simulink model "PVAndBatteryIntegratedPlantForBlackStart"  (R2025b)
settings: Solver=FixedStepAuto  StartTime=0.0  StopTime=tsim  FixedStep=1e-6  RelTol=1e-9  AbsTol=1e-7
InitFcn:
  | %% Black Start Sequence
  | t0 = 0; % Battery IBR initial time
  | t1 = 0.15; % PV IBR initial time
  | t2 = 0.5; % Two IBR sync time
  | t3 = 0.8; % Additional motor load connect
  | t4 = 1.1; % Grid reconnection
  | tsim = 1.5; % Total simulation time
  | 
  | %% initialize
  | Vdc = 400;
  | Vnom = 100;
  | Prated = 10000;
  | Qrated = 0;
  | Srated = sqrt(Prated^2+Qrated^2);
  | wnom = 2*pi*60;
  | fnom = 60;
  | Vminpu = 0.95;
  | 
  | kv = Vnom;
  | ki = 3*Vnom/Srated;
  | 
  | dwmax = 0.5*2*pi;
  | trisemax = 0.1;
  | 
  | C = 1/sqrt(2)/Vminpu^2/dwmax;
  | L = 1/C/wnom^2;
  | tau = C/kv/ki;
  | epsilon = sqrt(L/C);
  | ksy = 3/2/trisemax;
  | 
  | V_voc_1 = 0;
  | V_voc_2 = 0;
  | 
  | % filter
  | Rf = 0.05;
  | Lf = 500e-6;
  | % pwm
  | fsw = 10e3;
  | % simulation
  | Ts = 1e-6;
  | 
  | % load
  | Rl = 3*Vnom^2/Prated;
  | Rl1 = Rl;
  | Rl2 = 2*Rl;
  | Rl3 = 20*Rl;
  | % grid
  | Rg = 0.05;
  | Lg = 50e-6;
  | 
  | % DCDC converter
  | Kp_V = 1;
  | Ki_V = 0.02;
  | Imax = 110;
  | Kp_I = 0.0001;
  | Ki_I = 1;
  | Vcmax = 1;
undefined symbols (not defined in the file): alpha, C_voc, Diode_class, Half_BridgeConverter_class, L_voc, Ll, Mosfet_class, PWMGenerator_DC_DC__class, R_voc, Three_PhaseBreaker_class, Three_PhaseSource_class, Three_PhaseTransformer_2_class, Three_PhaseV_IMeasuremen_class
libraries: nesl_utility x69, ee_lib x49, fl_lib x36, mcbeeMathTransformLib x9, simulink x6, spsParallelRLCBranchLib x3, eePwmGeneratorTwoLevel x2, spsControlledCurrentSourceLib x2, elec_conv_HighZElecRef x2, slpidlib x2, spsSecondOrderFilterLib x1, spsCurrentMeasurementLib x1
(part 3 of 4)

== system PVAndBatteryIntegratedPlantForBlackStart/PV Inverter /PV Array ==
  S : Inport
  TempC : Inport  Port=2
  CSns : fl_lib/Electrical/Electrical Sensors/Current Sensor
  SC : ee_lib/Sources/Solar Cell  prm=ee.enum.sources.solar_cell_prm.datasheet  Isc=11.31 A  Voc=0.66071 V  Is=1e-6 A  Is2=0 A  Iph=11.31 A  Ir0=1000 W/m^2  ec=1.5  N2=2  Rs=0.0033987 Ohm  Rp=2.559 Ohm  N_series=280  N_parallel=10  TIPH1=0 1/K  EG=1.11 eV  TXIS1=3  TXIS2=3  TRS1=0  TRP1=0  Tmeas=25 degC  TFIXED=25 degC  thermal_mass=100 J/K  initial_temperature=25 degC
  VSns : fl_lib/Electrical/Electrical Sensors/Voltage Sensor
  busM : BusCreator  Inputs=2
  i2s : nesl_utility/PS-Simulink Converter  PhysicalDomain=network_engine_domain  SubClassName=ps_output  LeftPortType=input  RightPortType=output  PseudoPeriodic=off  Frequencies=[]  VectorFormat=inherit  Unit=inherit  AffineConversion=off
  s2ps : nesl_utility/Simulink-PS Converter  PhysicalDomain=network_engine_domain  SubClassName=ps_input  LeftPortType=input  RightPortType=output  PseudoPeriodic=off  Frequencies=[]  NoiseDistribution=none  NoiseParameters=[]  Unit=W/m^2  AffineConversion=off  FilteringAndDerivatives=provide  SimscapeFilterOrder=1  InputFilterTimeConstant=0.001  UdotUserProvided=0
  termT : Terminator
  v2s : nesl_utility/PS-Simulink Converter  PhysicalDomain=network_engine_domain  SubClassName=ps_output  LeftPortType=input  RightPortType=output  PseudoPeriodic=off  Frequencies=[]  VectorFormat=inherit  Unit=inherit  AffineConversion=off
  + : PMIOPort  Side=Right
  - : PMIOPort  Port=2  Side=Right
  m : Outport  VectorParamsAs1DForOutWhenUnconnected=off
  wires:
  S/1 -> s2ps/1
  TempC/1 -> termT/1
  v2s/1 -> busM/1  "V_PV"
  busM/1 -> m/1
  i2s/1 -> busM/2  "I_PV"
  connections:
  CSns/RConn1 -- i2s/LConn1
  VSns/RConn1 -- v2s/LConn1
  CSns/RConn2 -- +/RConn1
  VSns/RConn2 -- SC/RConn1 -- -/RConn1
  s2ps/RConn1 -- SC/LConn1
  VSns/LConn1 -- SC/LConn2 -- CSns/LConn1

== system PVAndBatteryIntegratedPlantForBlackStart/PV Inverter /PWM Generator (DC-DC) ==
  D : Inport
  PWM Generator : eePwmGenerator/PWM Generator  CarrCount=Up  Tper=PWMGenerator_DC_DC__class(fsw).objParamMappingDerived.NewDerivedParam.Tper  Tdelay=0  Ts=Ts
  P : Outport  VectorParamsAs1DForOutWhenUnconnected=off
  wires:
  D/1 -> PWM Generator/1
  PWM Generator/1 -> P/1

== system PVAndBatteryIntegratedPlantForBlackStart/PV Inverter /Series RLC Branch ==
  Inductor : fl_lib/Electrical/Electrical Elements/Inductor  l=0.0006 H  r=0 Ohm  g=1e-9 1/Ohm  i_specify=off  i_priority=None  i=0 A  i_nominal_specify=off  i_nominal_value=1  i_nominal_unit=A  v_specify=off  v_priority=None  v=0 V  v_nominal_specify=off  v_nominal_value=1  v_nominal_unit=V  i_L_specify=on  i_L_priority=None  i_L=0 A  i_L_nominal_specify=off  i_L_nominal_value=1  i_L_nominal_unit=A
  Resistor : fl_lib/Electrical/Electrical Elements/Resistor  R=0.001 Ohm  i_specify=off  i_priority=None  i=0 A  i_nominal_specify=off  i_nominal_value=1  i_nominal_unit=A  v_specify=off  v_priority=None  v=0 V  v_nominal_specify=off  v_nominal_value=1  v_nominal_unit=V
  + : PMIOPort  Side=Left
  - : PMIOPort  Port=2  Side=Right
  connections:
  Inductor/LConn1 -- Resistor/RConn1
  +/RConn1 -- Resistor/LConn1
  Inductor/RConn1 -- -/RConn1

== system PVAndBatteryIntegratedPlantForBlackStart/PV Inverter /Series RLC Branch1 ==
  Capacitor : fl_lib/Electrical/Electrical Elements/Capacitor  c=0.01 F  r=1e-6 Ohm  g=0 1/Ohm  i_specify=off  i_priority=None  i=0 A  i_nominal_specify=off  i_nominal_value=1  i_nominal_unit=A  v_specify=off  v_priority=None  v=0 V  v_nominal_specify=off  v_nominal_value=1  v_nominal_unit=V  vc_specify=on  vc_priority=High  vc=Vdc V  vc_nominal_specify=off  vc_nominal_value=1  vc_nominal_unit=V
  Resistor : fl_lib/Electrical/Electrical Elements/Resistor  R=0.001 Ohm  i_specify=off  i_priority=None  i=0 A  i_nominal_specify=off  i_nominal_value=1  i_nominal_unit=A  v_specify=off  v_priority=None  v=0 V  v_nominal_specify=off  v_nominal_value=1  v_nominal_unit=V
  + : PMIOPort  Side=Left
  - : PMIOPort  Port=2  Side=Right
  connections:
  Capacitor/RConn1 -- -/RConn1
  +/RConn1 -- Resistor/LConn1
  Resistor/RConn1 -- Capacitor/LConn1

== system PVAndBatteryIntegratedPlantForBlackStart/PV Inverter /Series RLC Branch2 ==
  Capacitor : fl_lib/Electrical/Electrical Elements/Capacitor  c=0.001 F  r=1e-6 Ohm  g=0 1/Ohm  i_specify=off  i_priority=None  i=0 A  i_nominal_specify=off  i_nominal_value=1  i_nominal_unit=A  v_specify=off  v_priority=None  v=0 V  v_nominal_specify=off  v_nominal_value=1  v_nominal_unit=V  vc_specify=on  vc_priority=None  vc=0 V  vc_nominal_specify=off  vc_nominal_value=1  vc_nominal_unit=V
  Resistor : fl_lib/Electrical/Electrical Elements/Resistor  R=0.001 Ohm  i_specify=off  i_priority=None  i=0 A  i_nominal_specify=off  i_nominal_value=1  i_nominal_unit=A  v_specify=off  v_priority=None  v=0 V  v_nominal_specify=off  v_nominal_value=1  v_nominal_unit=V
  + : PMIOPort  Side=Left
  - : PMIOPort  Port=2  Side=Right
  connections:
  Capacitor/RConn1 -- -/RConn1
  +/RConn1 -- Resistor/LConn1
  Resistor/RConn1 -- Capacitor/LConn1

== system PVAndBatteryIntegratedPlantForBlackStart/PV Inverter /Three-Phase Breaker ==
  Circuit Breaker : ee_lib/Switches & Breakers/Circuit Breaker (Three-Phase)  R_closed=0.001 Ohm  G_open=Three_PhaseBreaker_class('open',1000000,Inf,t1,'off').objParamMappingDerived.NewDerivedParam.G_open 1/Ohm  threshold=0.5 V  breaker_behavior=ee.enum.switches.breakerBehavior.zeroCrossingEnable
      settings: InternalSimscapePortConfiguration="{\"Bottom\":[],\"Left\":[{\"id\":\"vT\",\"label\":\"vT\",\"type\":\"input\"},{\"id\":\"a1\",\"label\":\"a1\",\"type\":\"foundation.electrical.electrical\"},{\"id\":\"b1\",\"label\":\"b1\",\"type\":\"foundation.electrical.electrical\"},{\"id\":\"c1\",\"label\":\"c1\",\"type\":\"foundation.electrical.electrical\"}],\"Right\":[{\"id\":\"a2\",\"label\":\"a2\",\"type\":\"foundation.electrical.electrical\"},{\"id\":\"b2\",\"label\":\"b2\",\"type\":\"foundation.electrical.electrical\"},{\"id\":\"c2\",\"label\":\"c2\",\"type\":\"foundation.electrical.electrical\"}],\"Top\":[]}"
  com : Subsystem
  A : PMIOPort  Side=Left
  B : PMIOPort  Port=2  Side=Left
  C : PMIOPort  Port=3  Side=Left
  a : PMIOPort  Port=4  Side=Right
  b : PMIOPort  Port=5  Side=Right
  c : PMIOPort  Port=6  Side=Right
  connections:
  Circuit Breaker/LConn1 -- com/RConn1
  Circuit Breaker/LConn2 -- A/RConn1
  Circuit Breaker/LConn3 -- B/RConn1
  Circuit Breaker/LConn4 -- C/RConn1
  Circuit Breaker/RConn1 -- a/RConn1
  Circuit Breaker/RConn2 -- b/RConn1
  Circuit Breaker/RConn3 -- c/RConn1

== system PVAndBatteryIntegratedPlantForBlackStart/PV Inverter /VOC Control ==
  Ifb : Inport
  P : Inport  Port=2
  Q : Inport  Port=3
  Constant : Constant  Value=0
  Inverse Clarke Transform : mcbeeMathTransformLib/Inverse Clarke Transform  PowerInvariant=off  UseWithEmbedded=off  PhaseInput=Two inputs
      settings: LibrarySourceBlock=|
      | ee_sl_lib/Mathematical
      | Transforms/Inverse
      | Clarke Transform
  Memory : Memory
  Memory1 : Memory
  Mux1 : Mux  Inputs=3
  Mux2 : Mux  Inputs=2
  Scope2 : Scope  NumInputPorts=6
      settings: ActiveDisplayYMinimum=-1297.23542  ActiveDisplayYMaximum=1334.98027
  Subsystem : Subsystem
  VOC_DE : Subsystem
  Vref : Outport
  tag scope: V_albe_inv_2=global
  wires:
  Mux2/1 -> [V_albe_inv_2]
  Q/1 -> Subsystem/3(Q)
  P/1 -> Subsystem/2(P)
  Subsystem/1(u) -> VOC_DE/1(u), Scope2/2
  Constant/1 -> Mux1/3
  VOC_DE/2(vbe) -> Memory1/1, Mux2/2, Mux1/2, Scope2/4
  VOC_DE/1(val) -> Mux1/1, Scope2/3, Memory/1, Mux2/1
  Inverse Clarke Transform/1 -> Scope2/6, Vref/1
  Ifb/1 -> Scope2/1, Subsystem/1(If)
  Mux1/1 -> Inverse Clarke Transform/1, Scope2/5
  Memory/1 -> Subsystem/4(val)
  Memory1/1 -> Subsystem/5(vbe)

== system PVAndBatteryIntegratedPlantForBlackStart/PV Inverter /Voltage Measurement ==
  PS-Simulink Converter : nesl_utility/PS-Simulink Converter  PhysicalDomain=network_engine_domain  SubClassName=ps_output  LeftPortType=input  RightPortType=output  PseudoPeriodic=off  Frequencies=[]  VectorFormat=1-D array  Unit=V  AffineConversion=off
  Voltage Sensor : fl_lib/Electrical/Electrical Sensors/Voltage Sensor
  + : PMIOPort  Side=Left
  - : PMIOPort  Port=2  Side=Left
  v : Outport  VectorParamsAs1DForOutWhenUnconnected=off
  wires:
  PS-Simulink Converter/1 -> v/1
  connections:
  PS-Simulink Converter/LConn1 -- Voltage Sensor/RConn1
  -/RConn1 -- Voltage Sensor/RConn2
  +/RConn1 -- Voltage Sensor/LConn1

== system PVAndBatteryIntegratedPlantForBlackStart/PV Inverter /inv ==
  Current and Voltage Sensor (Three-Phase) : ee_lib/Sensors & Transducers/Current and Voltage Sensor (Three-Phase)  vMeasurementType=2  outputUnit=2  SRated=100000000 V*A  VRated=500000 V  I_specify=off  I_priority=None  I=[ 0 0 0 ] A  I_nominal_specify=off  I_nominal_value=1  I_nominal_unit=A  V_specify=off  V_priority=None  V=[ 0 0 0 ] V  V_nominal_specify=off  V_nominal_value=1  V_nominal_unit=V
      settings: InternalSimscapePortConfiguration="{\"Bottom\":[],\"Left\":[{\"id\":\"a1\",\"label\":\"a1\",\"type\":\"foundation.electrical.electrical\"},{\"id\":\"b1\",\"label\":\"b1\",\"type\":\"foundation.electrical.electrical\"},{\"id\":\"c1\",\"label\":\"c1\",\"type\":\"foundation.electrical.electrical\"}],\"Right\":[{\"id\":\"V_output\",\"label\":\"V\",\"type\":\"output\"},{\"id\":\"I_output\",\"label\":\"I\",\"type\":\"output\"},{\"id\":\"a2\",\"label\":\"a2\",\"type\":\"foundation.electrical.electrical\"},{\"id\":\"b2\",\"label\":\"b2\",\"type\":\"foundation.electrical.electrical\"},{\"id\":\"c2\",\"label\":\"c2\",\"type\":\"foundation.electrical.electrical\"}],\"Top\":[]}"
  Igain : Gain  Gain=Three_PhaseV_IMeasuremen_class('phase-to-ground','yes','off','off','off',100000000,500000).objParamMappingDerived.NewDerivedParam.IG
  PS-Simulink Converter : nesl_utility/PS-Simulink Converter  PhysicalDomain=network_engine_domain  SubClassName=ps_output  LeftPortType=input  RightPortType=output  PseudoPeriodic=off  Frequencies=[]  VectorFormat=1-D array  Unit=1  AffineConversion=off
  PS-Simulink Converter1 : nesl_utility/PS-Simulink Converter  PhysicalDomain=network_engine_domain  SubClassName=ps_output  LeftPortType=input  RightPortType=output  PseudoPeriodic=off  Frequencies=[]  VectorFormat=1-D array  Unit=1  AffineConversion=off
  Vgain : Gain  Gain=Three_PhaseV_IMeasuremen_class('phase-to-ground','yes','off','off','off',100000000,500000).objParamMappingDerived.NewDerivedParam.VG
  A : PMIOPort  Side=Left
  B : PMIOPort  Port=2  Side=Left
  C : PMIOPort  Port=3  Side=Left
  a : PMIOPort  Port=4  Side=Right
  b : PMIOPort  Port=5  Side=Right
  c : PMIOPort  Port=6  Side=Right
  Vabc : Outport  VectorParamsAs1DForOutWhenUnconnected=off
  Iabc : Outport  Port=2  VectorParamsAs1DForOutWhenUnconnected=off
  wires:
  Igain/1 -> Iabc/1
  Vgain/1 -> Vabc/1
  PS-Simulink Converter1/1 -> Igain/1
  PS-Simulink Converter/1 -> Vgain/1
  connections:
  Current and Voltage Sensor (Three-Phase)/RConn1 -- PS-Simulink Converter/LConn1
  Current and Voltage Sensor (Three-Phase)/RConn2 -- PS-Simulink Converter1/LConn1
  Current and Voltage Sensor (Three-Phase)/RConn5 -- c/RConn1
  Current and Voltage Sensor (Three-Phase)/RConn4 -- b/RConn1
  Current and Voltage Sensor (Three-Phase)/RConn3 -- a/RConn1
  Current and Voltage Sensor (Three-Phase)/LConn3 -- C/RConn1
  Current and Voltage Sensor (Three-Phase)/LConn1 -- A/RConn1
  Current and Voltage Sensor (Three-Phase)/LConn2 -- B/RConn1

== system PVAndBatteryIntegratedPlantForBlackStart/PV Inverter /inv1 ==
  Current and Voltage Sensor (Three-Phase) : ee_lib/Sensors & Transducers/Current and Voltage Sensor (Three-Phase)  vMeasurementType=2  outputUnit=2  SRated=100000000 V*A  VRated=500000 V  I_specify=off  I_priority=None  I=[ 0 0 0 ] A  I_nominal_specify=off  I_nominal_value=1  I_nominal_unit=A  V_specify=off  V_priority=None  V=[ 0 0 0 ] V  V_nominal_specify=off  V_nominal_value=1  V_nominal_unit=V
      settings: InternalSimscapePortConfiguration="{\"Bottom\":[],\"Left\":[{\"id\":\"a1\",\"label\":\"a1\",\"type\":\"foundation.electrical.electrical\"},{\"id\":\"b1\",\"label\":\"b1\",\"type\":\"foundation.electrical.electrical\"},{\"id\":\"c1\",\"label\":\"c1\",\"type\":\"foundation.electrical.electrical\"}],\"Right\":[{\"id\":\"V_output\",\"label\":\"V\",\"type\":\"output\"},{\"id\":\"I_output\",\"label\":\"I\",\"type\":\"output\"},{\"id\":\"a2\",\"label\":\"a2\",\"type\":\"foundation.electrical.electrical\"},{\"id\":\"b2\",\"label\":\"b2\",\"type\":\"foundation.electrical.electrical\"},{\"id\":\"c2\",\"label\":\"c2\",\"type\":\"foundation.electrical.electrical\"}],\"Top\":[]}"
  Igain : Gain  Gain=Three_PhaseV_IMeasuremen_class('phase-to-ground','yes','off','off','off',100000000,500000).objParamMappingDerived.NewDerivedParam.IG
  PS-Simulink Converter : nesl_utility/PS-Simulink Converter  PhysicalDomain=network_engine_domain  SubClassName=ps_output  LeftPortType=input  RightPortType=output  PseudoPeriodic=off  Frequencies=[]  VectorFormat=1-D array  Unit=1  AffineConversion=off
  PS-Simulink Converter1 : nesl_utility/PS-Simulink Converter  PhysicalDomain=network_engine_domain  SubClassName=ps_output  LeftPortType=input  RightPortType=output  PseudoPeriodic=off  Frequencies=[]  VectorFormat=1-D array  Unit=1  AffineConversion=off
  Vgain : Gain  Gain=Three_PhaseV_IMeasuremen_class('phase-to-ground','yes','off','off','off',100000000,500000).objParamMappingDerived.NewDerivedParam.VG
  A : PMIOPort  Side=Left
  B : PMIOPort  Port=2  Side=Left
  C : PMIOPort  Port=3  Side=Left
  a : PMIOPort  Port=4  Side=Right
  b : PMIOPort  Port=5  Side=Right
  c : PMIOPort  Port=6  Side=Right
  Vabc : Outport  VectorParamsAs1DForOutWhenUnconnected=off
  Iabc : Outport  Port=2  VectorParamsAs1DForOutWhenUnconnected=off
  wires:
  Igain/1 -> Iabc/1
  Vgain/1 -> Vabc/1
  PS-Simulink Converter1/1 -> Igain/1
  PS-Simulink Converter/1 -> Vgain/1
  connections:
  Current and Voltage Sensor (Three-Phase)/RConn1 -- PS-Simulink Converter/LConn1
  Current and Voltage Sensor (Three-Phase)/RConn2 -- PS-Simulink Converter1/LConn1
  Current and Voltage Sensor (Three-Phase)/RConn5 -- c/RConn1
  Current and Voltage Sensor (Three-Phase)/RConn4 -- b/RConn1
  Current and Voltage Sensor (Three-Phase)/RConn3 -- a/RConn1
  Current and Voltage Sensor (Three-Phase)/LConn3 -- C/RConn1
  Current and Voltage Sensor (Three-Phase)/LConn1 -- A/RConn1
  Current and Voltage Sensor (Three-Phase)/LConn2 -- B/RConn1

== system PVAndBatteryIntegratedPlantForBlackStart/Three-Phase Breaker/com ==
  AND : Logic  Operator=NXOR  Inputs=5  IconShape=distinctive  AllPortsSameDT=off  OutDataTypeStr=boolean
  Data Type Conversion : DataTypeConversion  SaturateOnIntegerOverflow=off  RndMeth=Floor
  Simulink-PS Converter : nesl_utility/Simulink-PS Converter  PhysicalDomain=network_engine_domain  SubClassName=ps_input  LeftPortType=input  RightPortType=output  PseudoPeriodic=off  Frequencies=[]  NoiseDistribution=none  NoiseParameters=[]  Unit=1  AffineConversion=off  FilteringAndDerivatives=provide  SimscapeFilterOrder=1  InputFilterTimeConstant=0.001  UdotUserProvided=0
  Step : Step  Time=Three_PhaseBreaker_class('open',1000000,Inf,t4,'off').objParamMappingDerived.NewDerivedParam.switchTime1  SampleTime=0
  Step1 : Step  Time=Three_PhaseBreaker_class('open',1000000,Inf,t4,'off').objParamMappingDerived.NewDerivedParam.switchTime2  SampleTime=0
  Step2 : Step  Time=Three_PhaseBreaker_class('open',1000000,Inf,t4,'off').objParamMappingDerived.NewDerivedParam.switchTime3  SampleTime=0
  Step3 : Step  Time=Three_PhaseBreaker_class('open',1000000,Inf,t4,'off').objParamMappingDerived.NewDerivedParam.switchTime4  SampleTime=0
  Step4 : Step  Time=Three_PhaseBreaker_class('open',1000000,Inf,t4,'off').objParamMappingDerived.NewDerivedParam.switchTime5  SampleTime=0
  CB : PMIOPort  Side=Right
  wires:
  Data Type Conversion/1 -> Simulink-PS Converter/1
  Step4/1 -> AND/5
  AND/1 -> Data Type Conversion/1
  Step3/1 -> AND/4
  Step1/1 -> AND/2
  Step/1 -> AND/1
  Step2/1 -> AND/3
  connections:
  Simulink-PS Converter/RConn1 -- CB/RConn1

== system PVAndBatteryIntegratedPlantForBlackStart/Three-Phase Breaker1/com ==
  AND : Logic  Operator=NXOR  Inputs=5  IconShape=distinctive  AllPortsSameDT=off  OutDataTypeStr=boolean
  Data Type Conversion : DataTypeConversion  SaturateOnIntegerOverflow=off  RndMeth=Floor
  Simulink-PS Converter : nesl_utility/Simulink-PS Converter  PhysicalDomain=network_engine_domain  SubClassName=ps_input  LeftPortType=input  RightPortType=output  PseudoPeriodic=off  Frequencies=[]  NoiseDistribution=none  NoiseParameters=[]  Unit=1  AffineConversion=off  FilteringAndDerivatives=provide  SimscapeFilterOrder=1  InputFilterTimeConstant=0.001  UdotUserProvided=0
  Step : Step  Time=Three_PhaseBreaker_class('open',1000000,Inf,t2,'off').objParamMappingDerived.NewDerivedParam.switchTime1  SampleTime=0
  Step1 : Step  Time=Three_PhaseBreaker_class('open',1000000,Inf,t2,'off').objParamMappingDerived.NewDerivedParam.switchTime2  SampleTime=0
  Step2 : Step  Time=Three_PhaseBreaker_class('open',1000000,Inf,t2,'off').objParamMappingDerived.NewDerivedParam.switchTime3  SampleTime=0
  Step3 : Step  Time=Three_PhaseBreaker_class('open',1000000,Inf,t2,'off').objParamMappingDerived.NewDerivedParam.switchTime4  SampleTime=0
  Step4 : Step  Time=Three_PhaseBreaker_class('open',1000000,Inf,t2,'off').objParamMappingDerived.NewDerivedParam.switchTime5  SampleTime=0
  CB : PMIOPort  Side=Right
  wires:
  Data Type Conversion/1 -> Simulink-PS Converter/1
  Step4/1 -> AND/5
  AND/1 -> Data Type Conversion/1
  Step3/1 -> AND/4
  Step1/1 -> AND/2
  Step/1 -> AND/1
  Step2/1 -> AND/3
  connections:
  Simulink-PS Converter/RConn1 -- CB/RConn1

== system PVAndBatteryIntegratedPlantForBlackStart/Three-Phase Breaker2/com ==
  AND : Logic  Operator=NXOR  Inputs=5  IconShape=distinctive  AllPortsSameDT=off  OutDataTypeStr=boolean
  Data Type Conversion : DataTypeConversion  SaturateOnIntegerOverflow=off  RndMeth=Floor
  Simulink-PS Converter : nesl_utility/Simulink-PS Converter  PhysicalDomain=network_engine_domain  SubClassName=ps_input  LeftPortType=input  RightPortType=output  PseudoPeriodic=off  Frequencies=[]  NoiseDistribution=none  NoiseParameters=[]  Unit=1  AffineConversion=off  FilteringAndDerivatives=provide  SimscapeFilterOrder=1  InputFilterTimeConstant=0.001  UdotUserProvided=0
  Step : Step  Time=Three_PhaseBreaker_class('open',1000000000,Inf,t3,'off').objParamMappingDerived.NewDerivedParam.switchTime1  SampleTime=0
  Step1 : Step  Time=Three_PhaseBreaker_class('open',1000000000,Inf,t3,'off').objParamMappingDerived.NewDerivedParam.switchTime2  SampleTime=0
  Step2 : Step  Time=Three_PhaseBreaker_class('open',1000000000,Inf,t3,'off').objParamMappingDerived.NewDerivedParam.switchTime3  SampleTime=0
  Step3 : Step  Time=Three_PhaseBreaker_class('open',1000000000,Inf,t3,'off').objParamMappingDerived.NewDerivedParam.switchTime4  SampleTime=0
  Step4 : Step  Time=Three_PhaseBreaker_class('open',1000000000,Inf,t3,'off').objParamMappingDerived.NewDerivedParam.switchTime5  SampleTime=0
  CB : PMIOPort  Side=Right
  wires:
  Data Type Conversion/1 -> Simulink-PS Converter/1
  Step4/1 -> AND/5
  AND/1 -> Data Type Conversion/1
  Step3/1 -> AND/4
  Step1/1 -> AND/2
  Step/1 -> AND/1
  Step2/1 -> AND/3
  connections:
  Simulink-PS Converter/RConn1 -- CB/RConn1

== system PVAndBatteryIntegratedPlantForBlackStart/Three-Phase Breaker3/com ==
  AND : Logic  Operator=NXOR  Inputs=5  IconShape=distinctive  AllPortsSameDT=off  OutDataTypeStr=boolean
  Data Type Conversion : DataTypeConversion  SaturateOnIntegerOverflow=off  RndMeth=Floor
  Simulink-PS Converter : nesl_utility/Simulink-PS Converter  PhysicalDomain=network_engine_domain  SubClassName=ps_input  LeftPortType=input  RightPortType=output  PseudoPeriodic=off  Frequencies=[]  NoiseDistribution=none  NoiseParameters=[]  Unit=1  AffineConversion=off  FilteringAndDerivatives=provide  SimscapeFilterOrder=1  InputFilterTimeConstant=0.001  UdotUserProvided=0
  Step : Step  Time=Three_PhaseBreaker_class('open',1000000,Inf,t4,'off').objParamMappingDerived.NewDerivedParam.switchTime1  SampleTime=0
  Step1 : Step  Time=Three_PhaseBreaker_class('open',1000000,Inf,t4,'off').objParamMappingDerived.NewDerivedParam.switchTime2  SampleTime=0
  Step2 : Step  Time=Three_PhaseBreaker_class('open',1000000,Inf,t4,'off').objParamMappingDerived.NewDerivedParam.switchTime3  SampleTime=0
  Step3 : Step  Time=Three_PhaseBreaker_class('open',1000000,Inf,t4,'off').objParamMappingDerived.NewDerivedParam.switchTime4  SampleTime=0
  Step4 : Step  Time=Three_PhaseBreaker_class('open',1000000,Inf,t4,'off').objParamMappingDerived.NewDerivedParam.switchTime5  SampleTime=0
  CB : PMIOPort  Side=Right
  wires:
  Data Type Conversion/1 -> Simulink-PS Converter/1
  Step4/1 -> AND/5
  AND/1 -> Data Type Conversion/1
  Step3/1 -> AND/4
  Step1/1 -> AND/2
  Step/1 -> AND/1
  Step2/1 -> AND/3
  connections:
  Simulink-PS Converter/RConn1 -- CB/RConn1

== system PVAndBatteryIntegratedPlantForBlackStart/Battery Inverter/Inverter/Half-Bridge Converter ==
  " g " : Inport
  BL : Inport  Port=2
  Compare To Constant : simulink/Logic and Bit Operations/Compare To Constant  relop=<=  const=0.5  OutDataTypeStr=boolean
  Data Type Conversion : DataTypeConversion  OutDataTypeStr=double  SaturateOnIntegerOverflow=off  RndMeth=Floor
  Demux : Demux  Outputs=2
  Multiply : Product
  Simulink-PS Converter : nesl_utility/Simulink-PS Converter  PhysicalDomain=network_engine_domain  SubClassName=ps_input  LeftPortType=input  RightPortType=output  PseudoPeriodic=off  Frequencies=[]  NoiseDistribution=none  NoiseParameters=[]  Unit=1  AffineConversion=off  FilteringAndDerivatives=provide  SimscapeFilterOrder=1  InputFilterTimeConstant=0.001  UdotUserProvided=0
  Simulink-PS Converter1 : nesl_utility/Simulink-PS Converter  PhysicalDomain=network_engine_domain  SubClassName=ps_input  LeftPortType=input  RightPortType=output  PseudoPeriodic=off  Frequencies=[]  NoiseDistribution=none  NoiseParameters=[]  Unit=1  AffineConversion=off  FilteringAndDerivatives=provide  SimscapeFilterOrder=1  InputFilterTimeConstant=0.001  UdotUserProvided=0
  Two-Pulse Gate Multiplexer : ee_lib/Semiconductors & Converters/Converters/Two-Pulse Gate Multiplexer  port_option=ee.enum.controlport.ps
      settings: InternalSimscapePortConfiguration="{\"Bottom\":[],\"Left\":[{\"id\":\"G1_ps\",\"label\":\"G1\",\"type\":\"input\"},{\"id\":\"G2_ps\",\"label\":\"G2\",\"type\":\"input\"}],\"Right\":[{\"id\":\"p\",\"label\":\"G\",\"type\":\"foundation.electrical.four_phase\"}],\"Top\":[]}"
  Two-Quadrant Chopper : ee_lib/Semiconductors & Converters/Converters/Two-Quadrant Chopper  device_type=3  Vf=Half_BridgeConverter_class('Switching devices',0.001,1000000,Inf,0.001,1000000,Inf,0.001).objParamMappingDerived.NewDerivedParam.Vf V  Ron=Half_BridgeConverter_class('Switching devices',0.001,1000000,Inf,0.001,1000000,Inf,0.001).objParamMappingDerived.NewDerivedParam.Ron Ohm  Rds=0.001 Ohm  Goff=Half_BridgeConverter_class('Switching devices',0.001,1000000,Inf,0.001,1000000,Inf,0.001).objParamMappingDerived.NewDerivedParam.Goff 1/Ohm  Vgt=1 V  Vgt_off=-1 V  Ih=1 A  Vth=0.5 V  K=0  diode_param=2  diode_Vf=Half_BridgeConverter_class('Switching devices',0.001,1000000,Inf,0.001,1000000,Inf,0.001).objParamMappingDerived.NewDerivedParam.diode_Vf V  diode_Ron=Half_BridgeConverter_class('Switching devices',0.001,1000000,Inf,0.001,1000000,Inf,0.001).objParamMappingDerived.NewDerivedParam.diode_Ron Ohm  diode_Goff=Half_BridgeConverter_class('Switching devices',0.001,1000000,Inf,0.001,1000000,Inf,0.001).objParamMappingDerived.NewDerivedParam.diode_Goff 1/Ohm  diode_C=50 nF  diode_iRM=-235 A  diode_iF=300 A  diode_idot=-50 A/us  diode_trr_param=1  diode_trr_factor=3  diode_trr=15 us  diode_Qrr=1500 s*uA  snubber_type=0  Cs=Half_BridgeConverter_class('Switching devices',0.001,1000000,Inf,0.001,1000000,Inf,0.001).objParamMappingDerived.NewDerivedParam.Cs F  Rs=Half_BridgeConverter_class('Switching devices',0.001,1000000,Inf,0.001,1000000,Inf,0.001).objParamMappingDerived.NewDerivedParam.Rs Ohm
      settings: InternalSimscapePortConfiguration="{\"Bottom\":[],\"Left\":[{\"id\":\"G\",\"label\":\"G\",\"type\":\"foundation.electrical.four_phase\"},{\"id\":\"p1\",\"label\":\"1+\",\"type\":\"foundation.electrical.electrical\"},{\"id\":\"n1\",\"label\":\"1-\",\"type\":\"foundation.electrical.electrical\"}],\"Right\":[{\"id\":\"p2\",\"label\":\"2+\",\"type\":\"foundation.electrical.electrical\"},{\"id\":\"n2\",\"label\":\"2-\",\"type\":\"foundation.electrical.electrical\"}],\"Top\":[]}"
  + : PMIOPort  Side=Right
  - : PMIOPort  Port=2  Side=Right
  1 : PMIOPort  Port=3  Side=Left
  wires:
  Demux/2 -> Simulink-PS Converter1/1
  Demux/1 -> Simulink-PS Converter/1
  Multiply/1 -> Demux/1
  Data Type Conversion/1 -> Multiply/2
  Compare To Constant/1 -> Data Type Conversion/1
  BL/1 -> Compare To Constant/1
  " g "/1 -> Multiply/1
  connections:
  Simulink-PS Converter1/RConn1 -- Two-Pulse Gate Multiplexer/LConn2
  Two-Pulse Gate Multiplexer/RConn1 -- Two-Quadrant Chopper/LConn1
  Simulink-PS Converter/RConn1 -- Two-Pulse Gate Multiplexer/LConn1
  +/RConn1 -- Two-Quadrant Chopper/LConn2
  1/RConn1 -- Two-Quadrant Chopper/RConn1
  Two-Quadrant Chopper/LConn3 -- Two-Quadrant Chopper/RConn2 -- -/RConn1

== system PVAndBatteryIntegratedPlantForBlackStart/Battery Inverter/Inverter/Half-Bridge Converter1 ==
  " g " : Inport
  BL : Inport  Port=2
  Compare To Constant : simulink/Logic and Bit Operations/Compare To Constant  relop=<=  const=0.5  OutDataTypeStr=boolean
  Data Type Conversion : DataTypeConversion  OutDataTypeStr=double  SaturateOnIntegerOverflow=off  RndMeth=Floor
  Demux : Demux  Outputs=2
  Multiply : Product
  Simulink-PS Converter : nesl_utility/Simulink-PS Converter  PhysicalDomain=network_engine_domain  SubClassName=ps_input  LeftPortType=input  RightPortType=output  PseudoPeriodic=off  Frequencies=[]  NoiseDistribution=none  NoiseParameters=[]  Unit=1  AffineConversion=off  FilteringAndDerivatives=provide  SimscapeFilterOrder=1  InputFilterTimeConstant=0.001  UdotUserProvided=0
  Simulink-PS Converter1 : nesl_utility/Simulink-PS Converter  PhysicalDomain=network_engine_domain  SubClassName=ps_input  LeftPortType=input  RightPortType=output  PseudoPeriodic=off  Frequencies=[]  NoiseDistribution=none  NoiseParameters=[]  Unit=1  AffineConversion=off  FilteringAndDerivatives=provide  SimscapeFilterOrder=1  InputFilterTimeConstant=0.001  UdotUserProvided=0
  Two-Pulse Gate Multiplexer : ee_lib/Semiconductors & Converters/Converters/Two-Pulse Gate Multiplexer  port_option=ee.enum.controlport.ps
      settings: InternalSimscapePortConfiguration="{\"Bottom\":[],\"Left\":[{\"id\":\"G1_ps\",\"label\":\"G1\",\"type\":\"input\"},{\"id\":\"G2_ps\",\"label\":\"G2\",\"type\":\"input\"}],\"Right\":[{\"id\":\"p\",\"label\":\"G\",\"type\":\"foundation.electrical.four_phase\"}],\"Top\":[]}"
  Two-Quadrant Chopper : ee_lib/Semiconductors & Converters/Converters/Two-Quadrant Chopper  device_type=3  Vf=Half_BridgeConverter_class('Switching devices',0.001,1000000,Inf,0.001,1000000,Inf,0.001).objParamMappingDerived.NewDerivedParam.Vf V  Ron=Half_BridgeConverter_class('Switching devices',0.001,1000000,Inf,0.001,1000000,Inf,0.001).objParamMappingDerived.NewDerivedParam.Ron Ohm  Rds=0.001 Ohm  Goff=Half_BridgeConverter_class('Switching devices',0.001,1000000,Inf,0.001,1000000,Inf,0.001).objParamMappingDerived.NewDerivedParam.Goff 1/Ohm  Vgt=1 V  Vgt_off=-1 V  Ih=1 A  Vth=0.5 V  K=0  diode_param=2  diode_Vf=Half_BridgeConverter_class('Switching devices',0.001,1000000,Inf,0.001,1000000,Inf,0.001).objParamMappingDerived.NewDerivedParam.diode_Vf V  diode_Ron=Half_BridgeConverter_class('Switching devices',0.001,1000000,Inf,0.001,1000000,Inf,0.001).objParamMappingDerived.NewDerivedParam.diode_Ron Ohm  diode_Goff=Half_BridgeConverter_class('Switching devices',0.001,1000000,Inf,0.001,1000000,Inf,0.001).objParamMappingDerived.NewDerivedParam.diode_Goff 1/Ohm  diode_C=50 nF  diode_iRM=-235 A  diode_iF=300 A  diode_idot=-50 A/us  diode_trr_param=1  diode_trr_factor=3  diode_trr=15 us  diode_Qrr=1500 s*uA  snubber_type=0  Cs=Half_BridgeConverter_class('Switching devices',0.001,1000000,Inf,0.001,1000000,Inf,0.001).objParamMappingDerived.NewDerivedParam.Cs F  Rs=Half_BridgeConverter_class('Switching devices',0.001,1000000,Inf,0.001,1000000,Inf,0.001).objParamMappingDerived.NewDerivedParam.Rs Ohm
      settings: InternalSimscapePortConfiguration="{\"Bottom\":[],\"Left\":[{\"id\":\"G\",\"label\":\"G\",\"type\":\"foundation.electrical.four_phase\"},{\"id\":\"p1\",\"label\":\"1+\",\"type\":\"foundation.electrical.electrical\"},{\"id\":\"n1\",\"label\":\"1-\",\"type\":\"foundation.electrical.electrical\"}],\"Right\":[{\"id\":\"p2\",\"label\":\"2+\",\"type\":\"foundation.electrical.electrical\"},{\"id\":\"n2\",\"label\":\"2-\",\"type\":\"foundation.electrical.electrical\"}],\"Top\":[]}"
  + : PMIOPort  Side=Right
  - : PMIOPort  Port=2  Side=Right
  1 : PMIOPort  Port=3  Side=Left
  wires:
  Demux/2 -> Simulink-PS Converter1/1
  Demux/1 -> Simulink-PS Converter/1
  Multiply/1 -> Demux/1
  Data Type Conversion/1 -> Multiply/2
  Compare To Constant/1 -> Data Type Conversion/1
  BL/1 -> Compare To Constant/1
  " g "/1 -> Multiply/1
  connections:
  Simulink-PS Converter1/RConn1 -- Two-Pulse Gate Multiplexer/LConn2
  Two-Pulse Gate Multiplexer/RConn1 -- Two-Quadrant Chopper/LConn1
  Simulink-PS Converter/RConn1 -- Two-Pulse Gate Multiplexer/LConn1
  +/RConn1 -- Two-Quadrant Chopper/LConn2
  1/RConn1 -- Two-Quadrant Chopper/RConn1
  Two-Quadrant Chopper/LConn3 -- Two-Quadrant Chopper/RConn2 -- -/RConn1

== system PVAndBatteryIntegratedPlantForBlackStart/Battery Inverter/Inverter/Half-Bridge Converter2 ==
  " g " : Inport
  BL : Inport  Port=2
  Compare To Constant : simulink/Logic and Bit Operations/Compare To Constant  relop=<=  const=0.5  OutDataTypeStr=boolean
  Data Type Conversion : DataTypeConversion  OutDataTypeStr=double  SaturateOnIntegerOverflow=off  RndMeth=Floor
  Demux : Demux  Outputs=2
  Multiply : Product
  Simulink-PS Converter : nesl_utility/Simulink-PS Converter  PhysicalDomain=network_engine_domain  SubClassName=ps_input  LeftPortType=input  RightPortType=output  PseudoPeriodic=off  Frequencies=[]  NoiseDistribution=none  NoiseParameters=[]  Unit=1  AffineConversion=off  FilteringAndDerivatives=provide  SimscapeFilterOrder=1  InputFilterTimeConstant=0.001  UdotUserProvided=0
  Simulink-PS Converter1 : nesl_utility/Simulink-PS Converter  PhysicalDomain=network_engine_domain  SubClassName=ps_input  LeftPortType=input  RightPortType=output  PseudoPeriodic=off  Frequencies=[]  NoiseDistribution=none  NoiseParameters=[]  Unit=1  AffineConversion=off  FilteringAndDerivatives=provide  SimscapeFilterOrder=1  InputFilterTimeConstant=0.001  UdotUserProvided=0
  Two-Pulse Gate Multiplexer : ee_lib/Semiconductors & Converters/Converters/Two-Pulse Gate Multiplexer  port_option=ee.enum.controlport.ps
      settings: InternalSimscapePortConfiguration="{\"Bottom\":[],\"Left\":[{\"id\":\"G1_ps\",\"label\":\"G1\",\"type\":\"input\"},{\"id\":\"G2_ps\",\"label\":\"G2\",\"type\":\"input\"}],\"Right\":[{\"id\":\"p\",\"label\":\"G\",\"type\":\"foundation.electrical.four_phase\"}],\"Top\":[]}"
  Two-Quadrant Chopper : ee_lib/Semiconductors & Converters/Converters/Two-Quadrant Chopper  device_type=3  Vf=Half_BridgeConverter_class('Switching devices',0.001,1000000,Inf,0.001,1000000,Inf,0.001).objParamMappingDerived.NewDerivedParam.Vf V  Ron=Half_BridgeConverter_class('Switching devices',0.001,1000000,Inf,0.001,1000000,Inf,0.001).objParamMappingDerived.NewDerivedParam.Ron Ohm  Rds=0.001 Ohm  Goff=Half_BridgeConverter_class('Switching devices',0.001,1000000,Inf,0.001,1000000,Inf,0.001).objParamMappingDerived.NewDerivedParam.Goff 1/Ohm  Vgt=1 V  Vgt_off=-1 V  Ih=1 A  Vth=0.5 V  K=0  diode_param=2  diode_Vf=Half_BridgeConverter_class('Switching devices',0.001,1000000,Inf,0.001,1000000,Inf,0.001).objParamMappingDerived.NewDerivedParam.diode_Vf V  diode_Ron=Half_BridgeConverter_class('Switching devices',0.001,1000000,Inf,0.001,1000000,Inf,0.001).objParamMappingDerived.NewDerivedParam.diode_Ron Ohm  diode_Goff=Half_BridgeConverter_class('Switching devices',0.001,1000000,Inf,0.001,1000000,Inf,0.001).objParamMappingDerived.NewDerivedParam.diode_Goff 1/Ohm  diode_C=50 nF  diode_iRM=-235 A  diode_iF=300 A  diode_idot=-50 A/us  diode_trr_param=1  diode_trr_factor=3  diode_trr=15 us  diode_Qrr=1500 s*uA  snubber_type=0  Cs=Half_BridgeConverter_class('Switching devices',0.001,1000000,Inf,0.001,1000000,Inf,0.001).objParamMappingDerived.NewDerivedParam.Cs F  Rs=Half_BridgeConverter_class('Switching devices',0.001,1000000,Inf,0.001,1000000,Inf,0.001).objParamMappingDerived.NewDerivedParam.Rs Ohm
      settings: InternalSimscapePortConfiguration="{\"Bottom\":[],\"Left\":[{\"id\":\"G\",\"label\":\"G\",\"type\":\"foundation.electrical.four_phase\"},{\"id\":\"p1\",\"label\":\"1+\",\"type\":\"foundation.electrical.electrical\"},{\"id\":\"n1\",\"label\":\"1-\",\"type\":\"foundation.electrical.electrical\"}],\"Right\":[{\"id\":\"p2\",\"label\":\"2+\",\"type\":\"foundation.electrical.electrical\"},{\"id\":\"n2\",\"label\":\"2-\",\"type\":\"foundation.electrical.electrical\"}],\"Top\":[]}"
  + : PMIOPort  Side=Right
  - : PMIOPort  Port=2  Side=Right
  1 : PMIOPort  Port=3  Side=Left
  wires:
  Demux/2 -> Simulink-PS Converter1/1
  Demux/1 -> Simulink-PS Converter/1
  Multiply/1 -> Demux/1
  Data Type Conversion/1 -> Multiply/2
  Compare To Constant/1 -> Data Type Conversion/1
  BL/1 -> Compare To Constant/1
  " g "/1 -> Multiply/1
  connections:
  Simulink-PS Converter1/RConn1 -- Two-Pulse Gate Multiplexer/LConn2
  Two-Pulse Gate Multiplexer/RConn1 -- Two-Quadrant Chopper/LConn1
  Simulink-PS Converter/RConn1 -- Two-Pulse Gate Multiplexer/LConn1
  +/RConn1 -- Two-Quadrant Chopper/LConn2
  1/RConn1 -- Two-Quadrant Chopper/RConn1
  Two-Quadrant Chopper/LConn3 -- Two-Quadrant Chopper/RConn2 -- -/RConn1

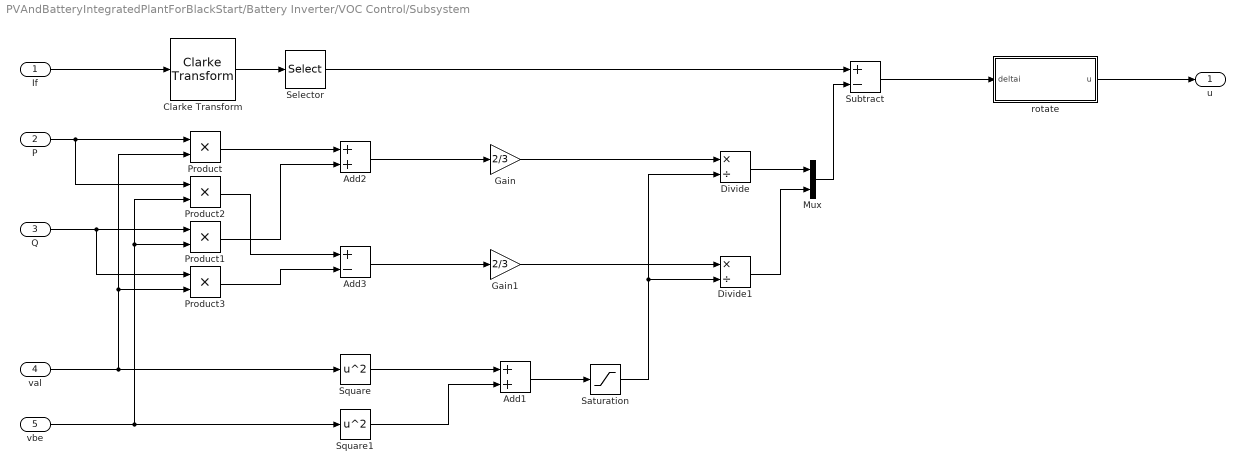
== system PVAndBatteryIntegratedPlantForBlackStart/Battery Inverter/VOC Control/Subsystem ==
  If : Inport
  P : Inport  Port=2
  Q : Inport  Port=3
  val : Inport  Port=4
  vbe : Inport  Port=5
  Add1 : Sum
  Add2 : Sum
  Add3 : Sum  Inputs=+-
  Clarke Transform : mcbeeMathTransformLib/Clarke Transform  PowerInvariant=off  UseWithEmbedded=off  PhaseInput=Two inputs
      settings: LibrarySourceBlock=|
      | ee_sl_lib/Mathematical
      | Transforms/Clarke Transform
  Divide : Product  Inputs=*/
  Divide1 : Product  Inputs=*/
  Gain : Gain  Gain=2/3
  Gain1 : Gain  Gain=2/3
  Mux : Mux  Inputs=2
  Product{,1..3} (4 alike) : Product
  Saturation : Saturate  UpperLimit=inf  LowerLimit=1e-9
  Selector : Selector  InputPortWidth=3  IndexOptions=Index vector (dialog)  Indices=[1 2]  OutputSizes=1
  Square : Math  Operator=square
  Square1 : Math  Operator=square
  Subtract : Sum  Inputs=+-
  rotate : Subsystem
  u : Outport
  wires:
  Clarke Transform/1 -> Selector/1
  If/1 -> Clarke Transform/1
  val/1 -> Product3/2, Product/2, Square/1
  vbe/1 -> Product2/2, Product1/2, Square1/1
  Square/1 -> Add1/1
  Square1/1 -> Add1/2
  Selector/1 -> Subtract/1
  Add1/1 -> Saturation/1
  P/1 -> Product2/1, Product/1
  Q/1 -> Product3/1, Product1/1
  Product/1 -> Add2/1
  Product1/1 -> Add2/2
  Add2/1 -> Gain/1
  Gain/1 -> Divide/1
  Saturation/1 -> Divide/2, Divide1/2
  Product2/1 -> Add3/1
  Product3/1 -> Add3/2
  Add3/1 -> Gain1/1
  Gain1/1 -> Divide1/1
  Divide/1 -> Mux/1
  Divide1/1 -> Mux/2
  Mux/1 -> Subtract/2
  Subtract/1 -> rotate/1(deltai)
  rotate/1(u) -> u/1

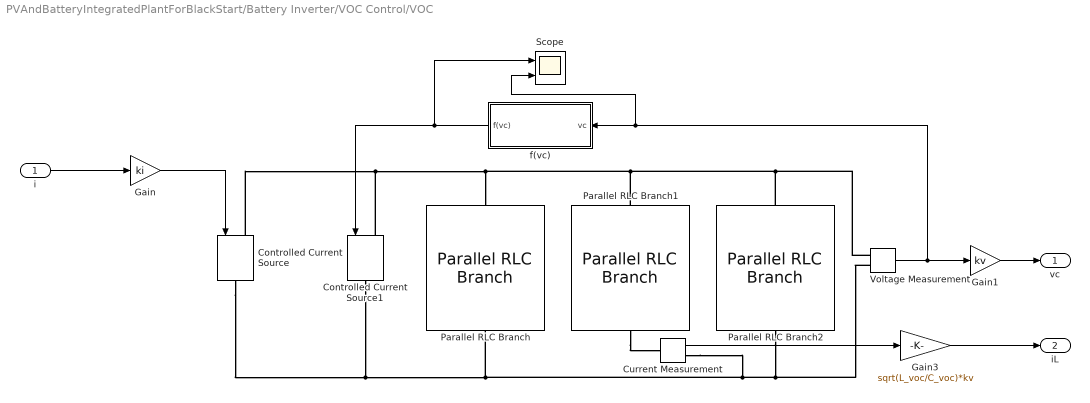
== system PVAndBatteryIntegratedPlantForBlackStart/Battery Inverter/VOC Control/VOC ==
  i : Inport
  Controlled Current Source : spsControlledCurrentSourceLib/Controlled Current Source  Initialize=off  Source_Type=AC  Amplitude=0  Phase=0  Frequency=0  Measurements=None
  Controlled Current Source1 : spsControlledCurrentSourceLib/Controlled Current Source  Initialize=off  Source_Type=AC  Amplitude=0  Phase=0  Frequency=0  Measurements=None
  Current Measurement : spsCurrentMeasurementLib/Current Measurement  PhasorSimulation=off  OutputType=Complex  PSBequivalent=0
  Gain : Gain  Gain=ki
  Gain1 : Gain  Gain=kv
  Gain3 : Gain  Gain=sqrt(L_voc/C_voc)*kv
  Parallel RLC Branch : spsParallelRLCBranchLib/Parallel RLC Branch  LConnTagsString=a  RConnTagsString=__new0  BranchType=R  Resistance=R_voc  Inductance=L_voc  SetiL0=off  InitialCurrent=0  Capacitance=C_voc  Setx0=off  InitialVoltage=0  Measurements=None
  Parallel RLC Branch1 : spsParallelRLCBranchLib/Parallel RLC Branch  LConnTagsString=a  RConnTagsString=__new0  BranchType=L  Resistance=R_voc  Inductance=L_voc  SetiL0=on  InitialCurrent=I_voc_1  Capacitance=C_voc  Setx0=off  InitialVoltage=0  Measurements=None
  Parallel RLC Branch2 : spsParallelRLCBranchLib/Parallel RLC Branch  LConnTagsString=a  RConnTagsString=__new0  BranchType=C  Resistance=R_voc  Inductance=L_voc  SetiL0=off  InitialCurrent=0  Capacitance=C_voc  Setx0=on  InitialVoltage=V_voc_1  Measurements=None
  Scope : Scope  NumInputPorts=2
      settings: ActiveDisplayYMinimum=-13.17018  ActiveDisplayYMaximum=13.17008
  Voltage Measurement : spsVoltageMeasurementLib/Voltage Measurement  PhasorSimulation=off  OutputType=Complex  PSBequivalent=0
  f(vc) : Subsystem
  vc : Outport
  iL : Outport  Port=2
  wires:
  i/1 -> Gain/1
  Voltage Measurement/1 -> Gain1/1, f(vc)/1(vc), Scope/2
  Gain/1 -> Controlled Current Source/1
  f(vc)/1(f(vc)) -> Scope/1, Controlled Current Source1/1
  Gain1/1 -> vc/1
  Gain3/1 -> iL/1
  Current Measurement/1 -> Gain3/1
  connections:
  Parallel RLC Branch2/RConn1 -- Voltage Measurement/LConn2 -- Current Measurement/RConn1 -- Controlled Current Source1/RConn1 -- Controlled Current Source/RConn1 -- Parallel RLC Branch/RConn1
  Controlled Current Source/LConn1 -- Controlled Current Source1/LConn1 -- Parallel RLC Branch/LConn1 -- Voltage Measurement/LConn1 -- Parallel RLC Branch2/LConn1 -- Parallel RLC Branch1/LConn1
  Parallel RLC Branch1/RConn1 -- Current Measurement/LConn1

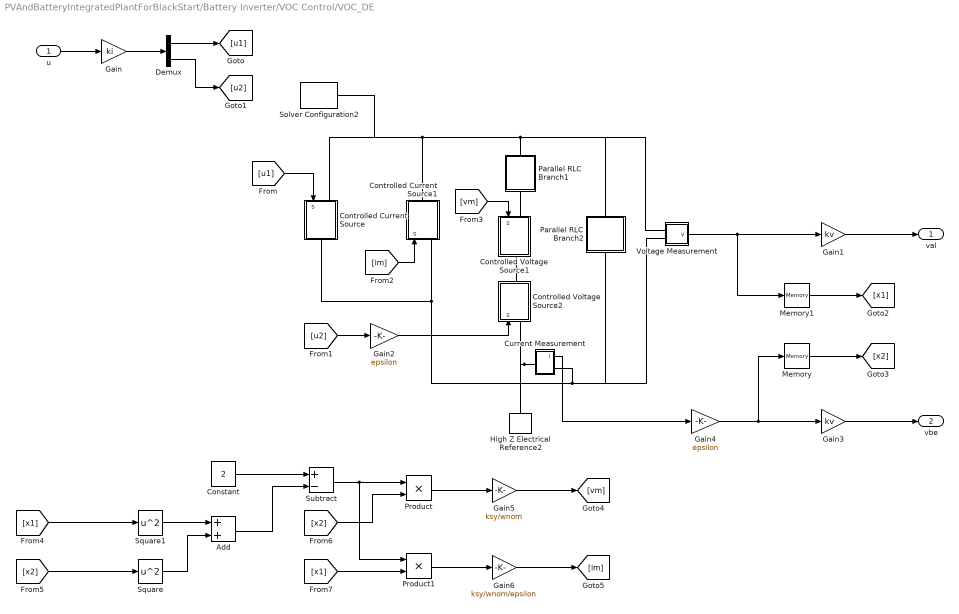
== system PVAndBatteryIntegratedPlantForBlackStart/Battery Inverter/VOC Control/VOC_DE ==
  u : Inport
  Add : Sum
  Constant : Constant  Value=2
  Controlled Current Source : Subsystem
      settings: OpenFcn=elec.conv.unmask(gcb);
  Controlled Current Source1 : Subsystem
      settings: OpenFcn=elec.conv.unmask(gcb);
  Controlled Voltage Source1 : Subsystem
      settings: OpenFcn=elec.conv.unmask(gcb);
  Controlled Voltage Source2 : Subsystem
      settings: OpenFcn=elec.conv.unmask(gcb);
  Current Measurement : Subsystem
      settings: OpenFcn=elec.conv.unmask(gcb);
  Demux : Demux  Outputs=2
  Gain : Gain  Gain=ki
  Gain1 : Gain  Gain=kv
  Gain2 : Gain  Gain=epsilon
  Gain3 : Gain  Gain=kv
  Gain4 : Gain  Gain=epsilon
  Gain5 : Gain  Gain=ksy/wnom
  Gain6 : Gain  Gain=ksy/wnom/epsilon
  High Z Electrical Reference2 : elec_conv_HighZElecRef/High Z Electrical Reference  SystemSampleTime=-1  VariantActivationTime=update diagram  EmptyChoice=off  PassThrough=off  PassThroughVariantControl=(default)  EmptyChoiceVariantControl=(default)  AllowFlexibleInterface=on  Latency=0  AutoFrameSizeCalculation=off
  Memory : Memory
  Memory1 : Memory
  Parallel RLC Branch1 : Subsystem
      settings: AttributesFormatString=\n  OpenFcn=elec.conv.unmask(gcb);
  Parallel RLC Branch2 : Subsystem
      settings: AttributesFormatString=\n  OpenFcn=elec.conv.unmask(gcb);
  Product : Product
  Product1 : Product
  Solver Configuration2 : nesl_utility/Solver Configuration  PhysicalDomain=network_engine_domain  SubClassName=solver  LeftPortType=input  RightPortType=generic  Tones=[]  Harmonics=[]  SimulateNoise=off  Profile=off  UseLocalSampling=off  EnableSwitchedLinearOptims=on  FrequencyDomain=off  UseCCode=off  RelTol=0.001  AbsTol=0.001  MinStep=1e-09  ToWorkspace=off  RevertToSquareIcSolve=off  NumHomotopyIterations=100  PhasorMode=off  PhasorModeNumHarmonics=1  ConsistencySolver=NEWTON_XTOL_AFTER_FTOL  IndexReductionMethod=DerivativeReplacement  DoDC=off  ResidualTolerance=1e-09  ConsistencyTolSource=GLOBAL  ConsistencyAbsTol=0.001  ConsistencyRelTol=0.001  ConsistencyTolFactor=0.001  UseLocalSolver=off  LocalSolverChoice=NE_BACKWARD_EULER_ADVANCER  ResolveIndetEquations=on  FunctionEvalNumThread=1  LocalSolverSampleTime=1e-6  DoFixedCost=on  MaxNonlinIter=3  MaxModeIter=2  ComputeImpulses=off  ImpulseIterations=2  LinearAlgebra=auto  LinearAlgebraNumThread=0  EquationFormulation=NE_TIME_EF  DelaysMemoryBudget=1024  AutomaticFiltering=on  FilteringTimeConstant=0.001  PartitionStorageMethod=AS_NEEDED  PartitionMemoryBudget=1024  PartitionMethod=ROBUST  MultibodyUseLocalSolver=off  MultibodyLocalSolverChoice=ODE1  MultibodyLocalSolverSampleTime=0.001
  Square : Math  Operator=square
  Square1 : Math  Operator=square
  Subtract : Sum  Inputs=+-
  Voltage Measurement : Subsystem
      settings: OpenFcn=elec.conv.unmask(gcb);
  val : Outport
  vbe : Outport  Port=2
  wires:
  Memory1/1 -> [x1]
  Memory/1 -> [x2]
  [x2] -> Square/1
  [x1] -> Square1/1
  u/1 -> Gain/1
  Voltage Measurement/1(v) -> Gain1/1, Memory1/1
  Gain1/1 -> val/1
  Gain/1 -> Demux/1
  Demux/1 -> [u1]
  Demux/2 -> [u2]
  [u1] -> Controlled Current Source/1(s)
  [u2] -> Gain2/1
  Gain2/1 -> Controlled Voltage Source2/1(s)
  [im] -> Controlled Current Source1/1(s)
  [vm] -> Controlled Voltage Source1/1(s)
  Gain3/1 -> vbe/1
  Gain4/1 -> Gain3/1, Memory/1
  Current Measurement/1(i) -> Gain4/1
  Constant/1 -> Subtract/1
  Square1/1 -> Add/1
  Square/1 -> Add/2
  Add/1 -> Subtract/2
  Subtract/1 -> Product1/1, Product/1
  [x2] -> Product/2
  Product/1 -> Gain5/1
  Gain5/1 -> [vm]
  [x1] -> Product1/2
  Product1/1 -> Gain6/1
  Gain6/1 -> [im]
  connections:
  Controlled Current Source1/LConn1 -- Controlled Current Source/RConn1 -- Current Measurement/RConn1 -- Parallel RLC Branch2/RConn1 -- Voltage Measurement/LConn2
  Controlled Current Source/LConn1 -- Solver Configuration2/RConn1 -- Controlled Current Source1/RConn1 -- Parallel RLC Branch1/LConn1 -- Parallel RLC Branch2/LConn1 -- Voltage Measurement/LConn1
  Controlled Voltage Source1/LConn1 -- Parallel RLC Branch1/RConn1
  Controlled Voltage Source2/RConn1 -- Controlled Voltage Source1/RConn1
  Current Measurement/LConn1 -- High Z Electrical Reference2/LConn1 -- Controlled Voltage Source2/LConn1
